simulink library "STD_Signaling_Lib"  (R2020b)
settings: Solver=VariableStepAuto  StartTime=0.0  StopTime=10.0  RelTol=1e-3
settings Model: Creator=mtarek-a  LastModifiedBy=amohsen2

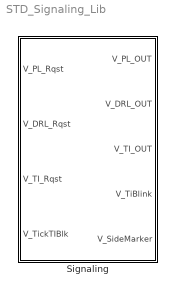
== system STD_Signaling_Lib ==
  Signaling : Subsystem

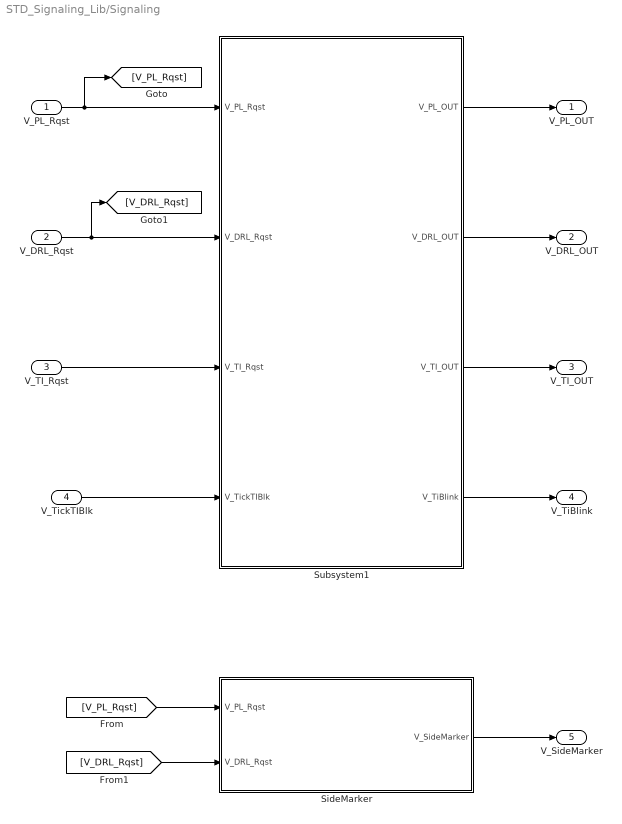
== system STD_Signaling_Lib/Signaling ==
  V_PL_Rqst : Inport
  V_DRL_Rqst : Inport  Port=2
  V_TI_Rqst : Inport  Port=3
  V_TickTIBlk : Inport  Port=4
  SideMarker : Subsystem  Description=|
      | requirement:
      | {S___EF_294 V00, S___EF_321 V00 }
  Subsystem1 : Subsystem
  V_PL_OUT : Outport
  V_DRL_OUT : Outport  Port=2
  V_TI_OUT : Outport  Port=3
  V_TiBlink : Outport  Port=4
  V_SideMarker : Outport  Port=5
  wires:
  V_PL_Rqst/1 -> Subsystem1/1(V_PL_Rqst), [V_PL_Rqst]
  V_DRL_Rqst/1 -> [V_DRL_Rqst], Subsystem1/2(V_DRL_Rqst)
  V_TI_Rqst/1 -> Subsystem1/3(V_TI_Rqst)
  V_TickTIBlk/1 -> Subsystem1/4(V_TickTIBlk)
  Subsystem1/3(V_TI_OUT) -> V_TI_OUT/1
  Subsystem1/4(V_TiBlink) -> V_TiBlink/1
  Subsystem1/1(V_PL_OUT) -> V_PL_OUT/1
  Subsystem1/2(V_DRL_OUT) -> V_DRL_OUT/1
  [V_PL_Rqst] -> SideMarker/1(V_PL_Rqst)
  [V_DRL_Rqst] -> SideMarker/2(V_DRL_Rqst)
  SideMarker/1(V_SideMarker) -> V_SideMarker/1

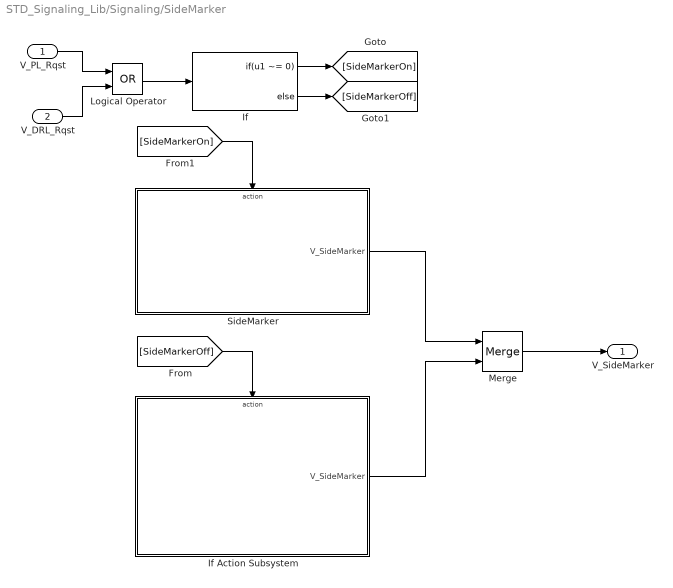
== system STD_Signaling_Lib/Signaling/SideMarker ==
  V_PL_Rqst : Inport
  V_DRL_Rqst : Inport  Port=2
  If : If  IfExpression=u1 ~= 0
  If Action Subsystem : Subsystem  TreatAsAtomicUnit=on
  Logical Operator : Logic  Operator=OR  AllPortsSameDT=off  OutDataTypeStr=boolean
  Merge : Merge
  SideMarker : Subsystem  TreatAsAtomicUnit=on
  V_SideMarker : Outport
  wires:
  Logical Operator/1 -> If/1
  V_PL_Rqst/1 -> Logical Operator/1
  V_DRL_Rqst/1 -> Logical Operator/2
  If/1 -> [SideMarkerOn]
  [SideMarkerOn] -> SideMarker/Action
  If/2 -> [SideMarkerOff]
  [SideMarkerOff] -> If Action Subsystem/Action
  Merge/1 -> V_SideMarker/1
  SideMarker/1(V_SideMarker) -> Merge/1
  If Action Subsystem/1(V_SideMarker) -> Merge/2

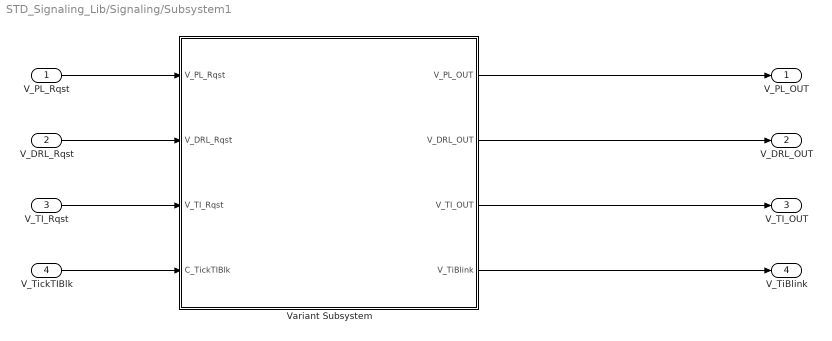
== system STD_Signaling_Lib/Signaling/Subsystem1 ==
  V_PL_Rqst : Inport
  V_DRL_Rqst : Inport  Port=2
  V_TI_Rqst : Inport  Port=3
  V_TickTIBlk : Inport  Port=4
  Variant Subsystem : Subsystem  Description=|  Variant=on  VariantActivationTime=code compile  AllowZeroVariantControls=on
      | requirement:
      | {S___EF_213 V00,S___EF_214 V00, S___EF_215 V00}
  V_PL_OUT : Outport
  V_DRL_OUT : Outport  Port=2
  V_TI_OUT : Outport  Port=3  OutDataTypeStr=boolean
  V_TiBlink : Outport  Port=4
  wires:
  V_TI_Rqst/1 -> Variant Subsystem/3(V_TI_Rqst)
  V_PL_Rqst/1 -> Variant Subsystem/1(V_PL_Rqst)
  V_DRL_Rqst/1 -> Variant Subsystem/2(V_DRL_Rqst)
  Variant Subsystem/2(V_DRL_OUT) -> V_DRL_OUT/1
  V_TickTIBlk/1 -> Variant Subsystem/4(C_TickTIBlk)
  Variant Subsystem/4(V_TiBlink) -> V_TiBlink/1
  Variant Subsystem/3(V_TI_OUT) -> V_TI_OUT/1
  Variant Subsystem/1(V_PL_OUT) -> V_PL_OUT/1

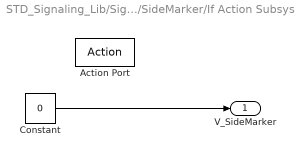
== system STD_Signaling_Lib/Signaling/SideMarker/If Action Subsystem ==
  Action Port : ActionPort  ActionPortLabel=else
  Constant : Constant  Value=0  OutDataTypeStr=Inherit: Inherit via back propagation
  V_SideMarker : Outport
  wires:
  Constant/1 -> V_SideMarker/1

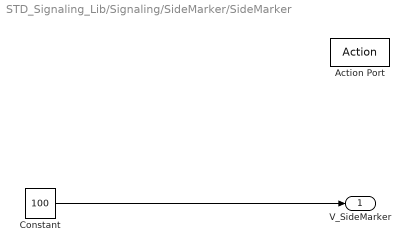
== system STD_Signaling_Lib/Signaling/SideMarker/SideMarker ==
  Action Port : ActionPort  ActionPortLabel=if(u1 ~= 0)
  Constant : Constant  Value=100  OutDataTypeStr=Inherit: Inherit via back propagation
  V_SideMarker : Outport
  wires:
  Constant/1 -> V_SideMarker/1

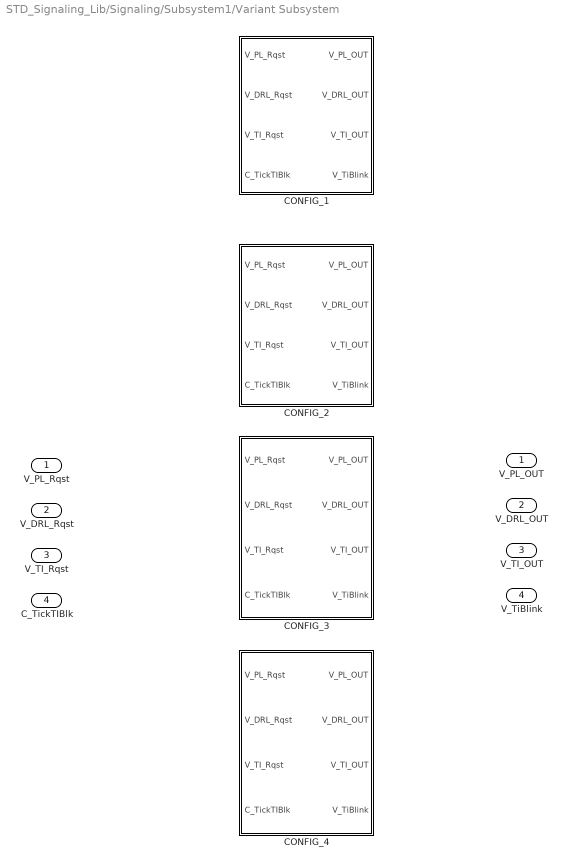
== system STD_Signaling_Lib/Signaling/Subsystem1/Variant Subsystem ==
  V_PL_Rqst : Inport
  V_DRL_Rqst : Inport  Port=2
  V_TI_Rqst : Inport  Port=3
  C_TickTIBlk : Inport  Port=4
  CONFIG_1 : Subsystem  Description=|  VariantControl=CONFIG_1
      | requirement:
      | {S___EF_192 V00,S___EF_219 V00,S___EF_228 V00,S___EF_232 V00,S___EF_233 V00,S___EF_234 V00}
  CONFIG_2 : Subsystem  Description=|  VariantControl=CONFIG_2
      | requirements:
      | {S___EF_216 V00,S___EF_220 V00,S___EF_239 V00,S___EF_240 V00,S___EF_241 V00, S___EF_242 V00 ,S___EF_243 V00,S___EF_244 V00, S___EF_245 V00 }
  CONFIG_3 : Subsystem  Description=|  VariantControl=CONFIG_3
      | requirements:
      | {S___EF_218 V00,S___EF_221 V00, S___EF_251 V00, S___EF_252 V00, S___EF_253 V00, S___EF_254 V00, S___EF_255 V00, S___EF_256 V00 , S___EF_257 V00, S___EF_258 V00}
  CONFIG_4 : Subsystem  Description=|  VariantControl=CONFIG_4
      | requirements:
      | {S___EF_217 V00,S___EF_222 V00, S___EF_264 V00, S___EF_265 V00, S___EF_266 V00, S___EF_268 V00, S___EF_268 V00, S___EF_270 V00, S___EF_269 V00, S___EF_271 V00, S___EF_275 V00 }
  V_PL_OUT : Outport
  V_DRL_OUT : Outport  Port=2
  V_TI_OUT : Outport  Port=3  OutDataTypeStr=boolean
  V_TiBlink : Outport  Port=4

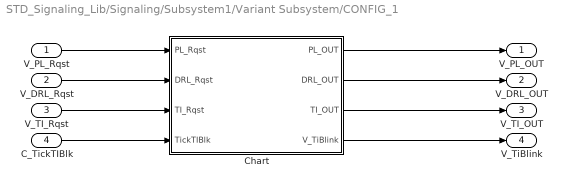
== system STD_Signaling_Lib/Signaling/Subsystem1/Variant Subsystem/CONFIG_1 ==
  V_PL_Rqst : Inport
  V_DRL_Rqst : Inport  Port=2
  V_TI_Rqst : Inport  Port=3
  C_TickTIBlk : Inport  Port=4
  Chart : Stateflow chart  TreatAsAtomicUnit=on
  V_PL_OUT : Outport
  V_DRL_OUT : Outport  Port=2
  V_TI_OUT : Outport  Port=3  OutDataTypeStr=boolean
  V_TiBlink : Outport  Port=4
  wires:
  V_TI_Rqst/1 -> Chart/3(TI_Rqst)
  C_TickTIBlk/1 -> Chart/4(TickTIBlk)
  Chart/1(PL_OUT) -> V_PL_OUT/1
  V_DRL_Rqst/1 -> Chart/2(DRL_Rqst)
  Chart/3(TI_OUT) -> V_TI_OUT/1
  Chart/4(V_TiBlink) -> V_TiBlink/1
  Chart/2(DRL_OUT) -> V_DRL_OUT/1
  V_PL_Rqst/1 -> Chart/1(PL_Rqst)

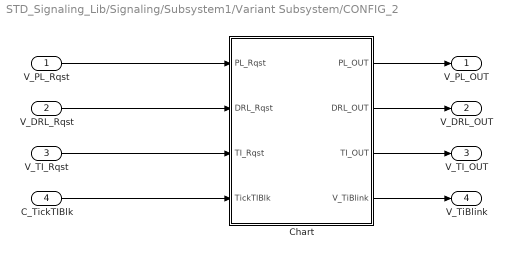
== system STD_Signaling_Lib/Signaling/Subsystem1/Variant Subsystem/CONFIG_2 ==
  V_PL_Rqst : Inport
  V_DRL_Rqst : Inport  Port=2
  V_TI_Rqst : Inport  Port=3
  C_TickTIBlk : Inport  Port=4
  Chart : Stateflow chart  TreatAsAtomicUnit=on
  V_PL_OUT : Outport
  V_DRL_OUT : Outport  Port=2
  V_TI_OUT : Outport  Port=3  OutDataTypeStr=boolean
  V_TiBlink : Outport  Port=4
  wires:
  V_PL_Rqst/1 -> Chart/1(PL_Rqst)
  Chart/2(DRL_OUT) -> V_DRL_OUT/1
  Chart/1(PL_OUT) -> V_PL_OUT/1
  Chart/4(V_TiBlink) -> V_TiBlink/1
  C_TickTIBlk/1 -> Chart/4(TickTIBlk)
  Chart/3(TI_OUT) -> V_TI_OUT/1
  V_TI_Rqst/1 -> Chart/3(TI_Rqst)
  V_DRL_Rqst/1 -> Chart/2(DRL_Rqst)

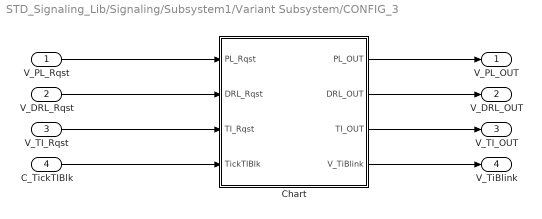
== system STD_Signaling_Lib/Signaling/Subsystem1/Variant Subsystem/CONFIG_3 ==
  V_PL_Rqst : Inport
  V_DRL_Rqst : Inport  Port=2
  V_TI_Rqst : Inport  Port=3
  C_TickTIBlk : Inport  Port=4
  Chart : Stateflow chart  TreatAsAtomicUnit=on
  V_PL_OUT : Outport
  V_DRL_OUT : Outport  Port=2
  V_TI_OUT : Outport  Port=3  OutDataTypeStr=boolean
  V_TiBlink : Outport  Port=4
  wires:
  Chart/3(TI_OUT) -> V_TI_OUT/1
  Chart/1(PL_OUT) -> V_PL_OUT/1
  C_TickTIBlk/1 -> Chart/4(TickTIBlk)
  V_PL_Rqst/1 -> Chart/1(PL_Rqst)
  V_DRL_Rqst/1 -> Chart/2(DRL_Rqst)
  V_TI_Rqst/1 -> Chart/3(TI_Rqst)
  Chart/2(DRL_OUT) -> V_DRL_OUT/1
  Chart/4(V_TiBlink) -> V_TiBlink/1

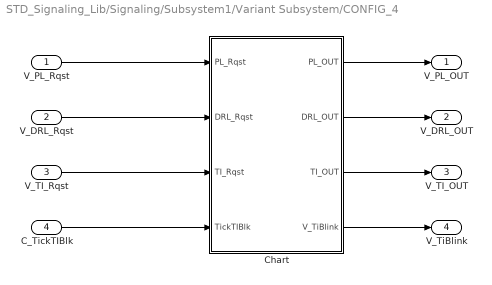
== system STD_Signaling_Lib/Signaling/Subsystem1/Variant Subsystem/CONFIG_4 ==
  V_PL_Rqst : Inport
  V_DRL_Rqst : Inport  Port=2
  V_TI_Rqst : Inport  Port=3
  C_TickTIBlk : Inport  Port=4
  Chart : Stateflow chart  TreatAsAtomicUnit=on
  V_PL_OUT : Outport
  V_DRL_OUT : Outport  Port=2
  V_TI_OUT : Outport  Port=3  OutDataTypeStr=boolean
  V_TiBlink : Outport  Port=4
  wires:
  V_DRL_Rqst/1 -> Chart/2(DRL_Rqst)
  C_TickTIBlk/1 -> Chart/4(TickTIBlk)
  Chart/1(PL_OUT) -> V_PL_OUT/1
  V_TI_Rqst/1 -> Chart/3(TI_Rqst)
  Chart/3(TI_OUT) -> V_TI_OUT/1
  V_PL_Rqst/1 -> Chart/1(PL_Rqst)
  Chart/2(DRL_OUT) -> V_DRL_OUT/1
  Chart/4(V_TiBlink) -> V_TiBlink/1

== stateflow chart STD_Signaling_Lib/Signaling/Subsystem1/Variant Subsystem/CONFIG_1/Chart ==
  state CONF1
    state TI [parallel]
      settings: executionOrder=1
      state OFF
        entry:
        TI_OUT=false;
        V_TiBlink=false;
      state ON
        entry:
        TI_OUT=true;
        V_TiBlink=true;
      state Blink
        entry:
        TI_OUT=false;
        V_TiBlink=true;
      (default) -> CONF1.TI.OFF
      Blink -> CONF1.TI.OFF [order 2] : [after(TickTIBlk,tick)]
      CONF1.TI.OFF -> ON : [TI_Rqst]
      Blink -> ON [order 1] : [TI_Rqst]
      ON -> Blink : [!TI_Rqst ]
    state DRL_PL [parallel]
      settings: executionOrder=2
      state OFF
        entry:
        PL_OUT=false;
        DRL_OUT=false;
      state PL
        entry:
        PL_OUT=true;
        DRL_OUT=false;
      state DRL
        entry:
        DRL_OUT=true;
        PL_OUT=false;
      (default) -> CONF1.DRL_PL.OFF
      CONF1.DRL_PL.OFF -> DRL [order 1] : [DRL_Rqst]
      (junction 31) -> CONF1.DRL_PL.OFF [order 2]
      PL -> CONF1.DRL_PL.OFF [order 2] : [ !PL_Rqst]
      CONF1.DRL_PL.OFF -> PL [order 2] : [PL_Rqst]
      (junction 31) -> PL [order 1] : [PL_Rqst]
      DRL -> (junction 31) : [!DRL_Rqst]
      PL -> DRL [order 1] : [DRL_Rqst]
  (default) -> CONF1
  data: PL_OUT output; DRL_OUT output; TI_OUT output; PL_Rqst input; DRL_Rqst input; TI_Rqst input; V_TiBlink output; TickTIBlk input

== stateflow chart STD_Signaling_Lib/Signaling/Subsystem1/Variant Subsystem/CONFIG_2/Chart ==
  state CONF2
    state OFF
      entry:
      TI_OUT=false;
      PL_OUT=false;
      DRL_OUT=false;
      V_TiBlink=false;
    state DRL
      entry:
      DRL_OUT=true;
      TI_OUT=false;
      PL_OUT=false;
      V_TiBlink=false;
    state TI
      state TI_S
        entry:
        TI_OUT=true;
        PL_OUT=false;
        DRL_OUT=false;
        V_TiBlink=true;
      state TI_S1
        entry:
        TI_OUT=false;
        PL_OUT=false;
        DRL_OUT=false;
        V_TiBlink=true;
      (default) -> TI_S
      TI_S1 -> TI_S [order 2] : [TI_Rqst]
      TI_S -> TI_S1 : [~TI_Rqst]
    state PL
      entry:
      PL_OUT=true;
      TI_OUT=false;
      DRL_OUT=false;
      V_TiBlink=false;
    (default) -> OFF
    OFF -> TI [order 1] : [TI_Rqst]
    (junction 60) -> OFF [order 3]
    OFF -> DRL [order 3] : [DRL_Rqst]
    DRL -> OFF [order 3] : [~DRL_Rqst]
    OFF -> PL [order 2] : [PL_Rqst]
    PL -> OFF [order 3] : [~PL_Rqst]
    (junction 60) -> DRL [order 2] : [DRL_Rqst]
    (junction 60) -> PL [order 1] : [PL_Rqst]
    TI_S1 -> (junction 60) [order 1] : [(~TI_Rqst &&(after(TickTIBlk,tick) )) ]
    PL -> DRL [order 2] : [DRL_Rqst]
    DRL -> TI [order 1] : [TI_Rqst]
    DRL -> PL [order 2] : [PL_Rqst]
    PL -> TI [order 1] : [TI_Rqst]
  (default) -> CONF2
  data: PL_Rqst input; DRL_Rqst input; TI_Rqst input; TickTIBlk input; PL_OUT output; DRL_OUT output; TI_OUT output; V_TiBlink output

== stateflow chart STD_Signaling_Lib/Signaling/Subsystem1/Variant Subsystem/CONFIG_3/Chart ==
  state CONF3
    state OFF
      entry:
      TI_OUT=false;
      PL_OUT=false;
      DRL_OUT=false;
      V_TiBlink=false;
    state DRL
      entry:
      DRL_OUT=true;
      TI_OUT=false;
      PL_OUT=false;
      V_TiBlink=false;
    state TI
      state TI_S
        entry:
        TI_OUT=true;
        PL_OUT=false;
        DRL_OUT=false;
        V_TiBlink=true;
      state PL_S
        state PL_off
          entry:
          PL_OUT=false;
          TI_OUT=false;
          DRL_OUT=false;
          V_TiBlink=true;
        state PL_on
          entry:
          TI_OUT=false;
          PL_OUT=true;
          DRL_OUT=false;
          V_TiBlink=true;
        (junction 87) -> PL_off [order 2]
        (junction 87) -> PL_on [order 1] : [(PL_Rqst) || (DRL_Rqst) ]
        PL_off -> PL_on : [(PL_Rqst) || (DRL_Rqst)]
        PL_on -> PL_off : [(~PL_Rqst) && (~DRL_Rqst) ]
      PL_S -> TI_S [order 2] : [TI_Rqst]
      TI_S -> (junction 87) : [~TI_Rqst]
    state PL
      entry:
      PL_OUT=true;
      TI_OUT=false;
      DRL_OUT=false;
      V_TiBlink=false;
    (default) -> OFF
    OFF -> TI_S [order 1] : [TI_Rqst]
    (junction 104) -> OFF [order 3]
    OFF -> DRL [order 2] : [DRL_Rqst]
    (junction 100) -> OFF [order 2]
    OFF -> PL [order 3] : [PL_Rqst]
    PL -> OFF [order 3] : [~PL_Rqst]
    DRL -> (junction 100) [order 2] : [~DRL_Rqst ]
    DRL -> TI_S [order 1] : [TI_Rqst]
    (junction 100) -> PL [order 1] : [PL_Rqst]
    (junction 104) -> DRL [order 1] : [DRL_Rqst]
    PL -> DRL [order 2] : [DRL_Rqst ]
    PL -> TI_S [order 1] : [TI_Rqst]
    PL_S -> (junction 104) [order 1] : [(~TI_Rqst && after(TickTIBlk,tick))]
    (junction 104) -> PL [order 2] : [PL_Rqst]
  (default) -> CONF3
  data: PL_Rqst input; DRL_Rqst input; TI_Rqst input; TickTIBlk input; PL_OUT output; DRL_OUT output; TI_OUT output; V_TiBlink output

== stateflow chart STD_Signaling_Lib/Signaling/Subsystem1/Variant Subsystem/CONFIG_4/Chart ==
  state CONF4
    state OFF
      entry:
      TI_OUT=false;
      PL_OUT=false;
      DRL_OUT=false;
      V_TiBlink=false;
    state DRL
      entry:
      DRL_OUT=true;
      TI_OUT=false;
      PL_OUT=false;
      V_TiBlink=false;
    state TI
      state TI_No_PL
        state TI_S
          entry:
          TI_OUT=true;
          PL_OUT=false;
          DRL_OUT=false;
          V_TiBlink=true;
        state TI_S1
          entry:
          TI_OUT=false;
          PL_OUT=false;
          DRL_OUT=false;
          V_TiBlink=true;
        TI_S1 -> TI_S [order 2] : [TI_Rqst]
        TI_S -> TI_S1 : [~TI_Rqst]
      state TI_And_PL
        state TIPL_S
          entry:
          TI_OUT=true;
          PL_OUT=true;
          DRL_OUT=false;
          V_TiBlink=true;
        state TIPL_S1
          entry:
          TI_OUT=false;
          PL_OUT=true;
          DRL_OUT=false;
          V_TiBlink=true;
        TIPL_S1 -> TIPL_S [order 1] : [TI_Rqst]
        TIPL_S -> TIPL_S1 : [~TI_Rqst]
      TI_And_PL -> (junction 73) : [(~PL_Rqst) && (~DRL_Rqst)]
      (junction 73) -> TI_S [order 1] : [TI_Rqst]
      (junction 73) -> TI_S1 [order 2]
      (junction 78) -> TIPL_S [order 1] : [TI_Rqst ]
      (junction 78) -> TIPL_S1 [order 2]
      TI_No_PL -> (junction 78) : [(PL_Rqst) || (DRL_Rqst)]
    state PL
      entry:
      PL_OUT=true;
      TI_OUT=false;
      DRL_OUT=false;
      V_TiBlink=false;
    (default) -> OFF
    OFF -> (junction 66) [order 1] : [TI_Rqst]
    (junction 15) -> OFF [order 3]
    OFF -> DRL [order 2] : [DRL_Rqst]
    (junction 34) -> OFF [order 2]
    OFF -> PL [order 3] : [PL_Rqst]
    PL -> OFF [order 3] : [~PL_Rqst]
    DRL -> (junction 66) [order 2] : [TI_Rqst]
    PL -> (junction 66) [order 1] : [TI_Rqst]
    (junction 66) -> TI_S [order 2]
    (junction 66) -> TIPL_S [order 1] : [(PL_Rqst) || (DRL_Rqst)]
    DRL -> (junction 34) [order 1] : [~DRL_Rqst]
    (junction 34) -> PL [order 1] : [PL_Rqst]
    (junction 15) -> DRL [order 1] : [DRL_Rqst]
    PL -> DRL [order 2] : [DRL_Rqst]
    TI_S1 -> (junction 15) [order 1] : [(~TI_Rqst && after(TickTIBlk,tick))]
    (junction 15) -> PL [order 2] : [PL_Rqst]
    TIPL_S1 -> (junction 15) [order 2] : [(~TI_Rqst && after(TickTIBlk,tick))]
  (default) -> CONF4
  data: PL_Rqst input; DRL_Rqst input; TI_Rqst input; TickTIBlk input; PL_OUT output; DRL_OUT output; TI_OUT output; V_TiBlink output
